simulink model "ASK_coerente"  (R2020a)
settings: Solver=VariableStepAuto  StartTime=0.0  StopTime=tsim  RelTol=1e-3
values from neighbouring files (symbols this model uses):
  Ac = 1    [init_vars.m]
  fc = 10e3    (= 10000)    [init_vars.m]
  fs = spb*rb    (= 100000)    [init_vars.m]
  ganho_int = rb    (= 1000)    [init_vars.m]
  lim = 0.5/2    (= 0.25)    [parte3ASK.m]    (also in parte3BPSK.m = 0; parte4.m = 0.5)
  rb = 1e3    (= 1000)    [init_vars.m]
  rng_seed = 5    [init_vars.m]
  spb = 100    [init_vars.m]
libraries: dspswit3 x2, commrandsrc3 x1, commchan3 x1, commfilt2 x1, dspsigops x1
settings Model: Creator=pedro  LastModifiedBy=pedro

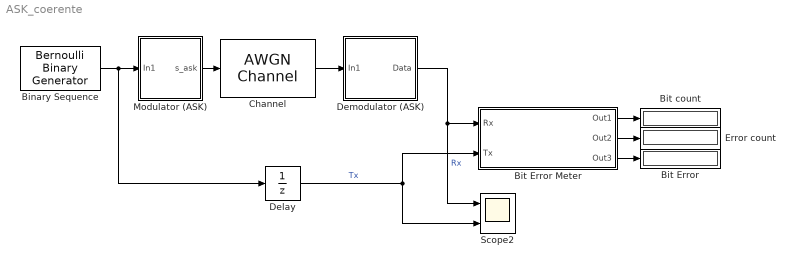
== system ASK_coerente ==
  Binary Sequence : commrandsrc3/Bernoulli Binary Generator  ProbabilityOfZero=0.5  SeedSource=Parameter  Seed=rng_seed  SampleTime=1/rb  SamplesPerFrame=1  OutputDataType=double  SimulateUsing=Interpreted execution
  Bit Error : Display
  Bit Error Meter : Subsystem
  Bit count : Display
  Channel : commchan3/AWGN Channel  InputProcessing=Columns as channels (frame based)  seed=rng_seed  noiseMode=Variance from mask  EbNodB=10  EsNodB=10  SNRdB=10  bitsPerSym=1  Ps=1  Tsym=1  variance=sigmaquadrado
  Delay : UnitDelay  SampleTime=1/rb  HasFrameUpgradeWarning=on
  Demodulator (ASK) : Subsystem
  Error count : Display
  Modulator (ASK) : Subsystem
  Scope2 : Scope  NumInputPorts=2
  wires:
  Binary Sequence/1 -> Delay/1, Modulator (ASK)/1(In1)
  Modulator (ASK)/1(s_ask) -> Channel/1
  Delay/1 -> Scope2/2, Bit Error Meter/2(Tx)  "Tx"
  Bit Error Meter/1(Out1) -> Bit count/1
  Bit Error Meter/2(Out2) -> Error count/1
  Bit Error Meter/3(Out3) -> Bit Error/1
  Demodulator (ASK)/1(Data) -> Bit Error Meter/1(Rx), Scope2/1  "Rx"
  Channel/1 -> Demodulator (ASK)/1(In1)

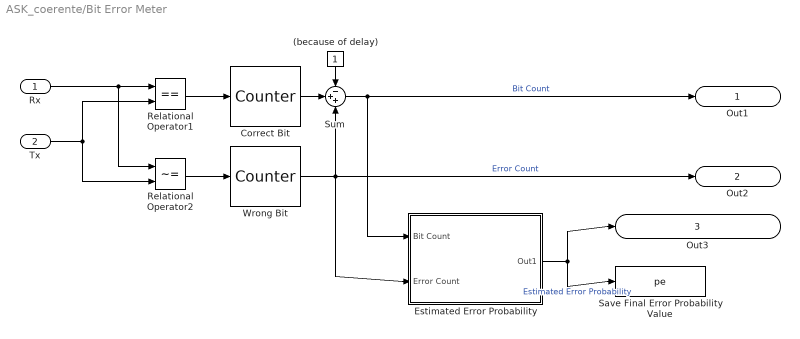
== system ASK_coerente/Bit Error Meter ==
  Rx : Inport
  Tx : Inport  Port=2
  (because of delay) : Constant
  Correct Bit : dspswit3/Counter  Direction=Up  CountEvent=Non-zero sample  CounterSize=32 bits  MaxCount=255  InitialCount=0  Output=Count  HitValue=32  ResetInput=off  SamplesPerFrame=1  Ts=1  CntDtype=uint32  HitDtype=Logical
  Estimated Error Probability : Subsystem
  Relational Operator1 : RelationalOperator  Operator===  OutDataTypeStr=boolean  RndMeth=Simplest
  Relational Operator2 : RelationalOperator  Operator=~=  OutDataTypeStr=boolean  RndMeth=Simplest
  Save Final Error Probability Value : ToWorkspace  VariableName=pe  SampleTime=-1
      settings: MaxDataPoints=1
  Sum : Sum  Inputs=-++
  Wrong Bit : dspswit3/Counter  Direction=Up  CountEvent=Non-zero sample  CounterSize=32 bits  MaxCount=255  InitialCount=0  Output=Count  HitValue=32  ResetInput=off  SamplesPerFrame=1  Ts=1  CntDtype=uint32  HitDtype=Logical
  Out1 : Outport
  Out2 : Outport  Port=2
  Out3 : Outport  Port=3
  wires:
  Relational Operator1/1 -> Correct Bit/1
  Correct Bit/1 -> Sum/2
  Rx/1 -> Relational Operator2/1, Relational Operator1/1
  Relational Operator2/1 -> Wrong Bit/1
  Sum/1 -> Estimated Error Probability/1(Bit Count), Out1/1  "Bit Count"
  Tx/1 -> Relational Operator2/2, Relational Operator1/2
  Wrong Bit/1 -> Estimated Error Probability/2(Error Count), Sum/3, Out2/1  "Error Count"
  (because of delay)/1 -> Sum/1
  Estimated Error Probability/1(Out1) -> Out3/1, Save Final Error Probability Value/1  "Estimated Error Probability"

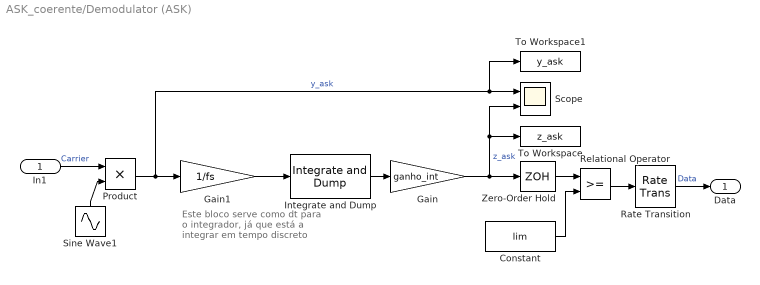
== system ASK_coerente/Demodulator (ASK) ==
  note: Este bloco serve como dt
      | para o integrador, já que está a integrar em tempo discreto
  In1 : Inport
  Constant : Constant  Value=lim
  Gain : Gain  Gain=ganho_int
  Gain1 : Gain  Gain=1/fs
  Integrate and Dump : commfilt2/Integrate and Dump  obssamples=spb  offsetsamples=1  nodump=on  roundingMode=Floor  overflowMode=off  outputDataTypeStr=Inherit: Same as accumulator  outputLastDataTypeStr=Inherit: Same as accumulator
  Product : Product
  Rate Transition : RateTransition  Integrity=off  OutPortSampleTime=1/rb
  Relational Operator : RelationalOperator  OutDataTypeStr=boolean  RndMeth=Simplest
  Scope : Scope  NumInputPorts=2
  Sine Wave1 : Sin  Amplitude=Ac  Frequency=2*pi*fc  SampleTime=1/fs
  To Workspace : ToWorkspace  VariableName=z_ask  SaveFormat=Timeseries  SampleTime=-1
  To Workspace1 : ToWorkspace  VariableName=y_ask  SaveFormat=Timeseries  SampleTime=-1
  Zero-Order Hold : ZeroOrderHold  SampleTime=1/rb
  Data : Outport
  wires:
  In1/1 -> Product/1  "Carrier"
  Product/1 -> To Workspace1/1, Scope/1, Gain1/1  "y_ask"
  Relational Operator/1 -> Rate Transition/1
  Sine Wave1/1 -> Product/2
  Integrate and Dump/1 -> Gain/1
  Constant/1 -> Relational Operator/2
  Zero-Order Hold/1 -> Relational Operator/1
  Gain/1 -> Scope/2, To Workspace/1, Zero-Order Hold/1  "z_ask"
  Rate Transition/1 -> Data/1  "Data"
  Gain1/1 -> Integrate and Dump/1

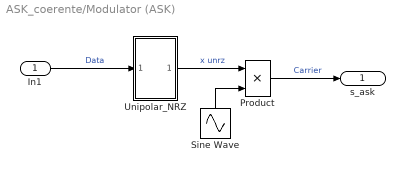
== system ASK_coerente/Modulator (ASK) ==
  In1 : Inport
  Product : Product
  Sine Wave : Sin  Amplitude=Ac  Frequency=2*pi*fc  SampleTime=1/fs
  Unipolar_NRZ : Subsystem  mask(unipolar_nrz){Rb=rb, Spb=spb}
      mask prompts: Rb "Binary Data Rate"; Spb "Samples per bit"
  s_ask : Outport
  wires:
  Sine Wave/1 -> Product/2
  Product/1 -> s_ask/1  "Carrier"
  Unipolar_NRZ/1(Out1) -> Product/1  "x unrz"
  In1/1 -> Unipolar_NRZ/1(In1)  "Data"

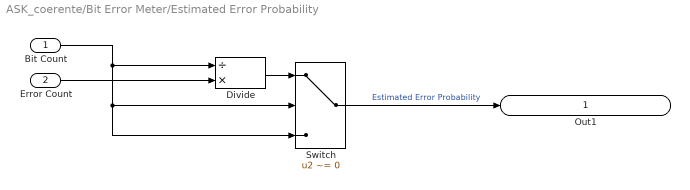
== system ASK_coerente/Bit Error Meter/Estimated Error Probability ==
  Bit Count : Inport
  Error Count : Inport  Port=2
  Divide : Product  Inputs=/*  OutDataTypeStr=double
  Switch : Switch  Criteria=u2 ~= 0
  Out1 : Outport
  wires:
  Bit Count/1 -> Divide/1, Switch/3, Switch/2
  Switch/1 -> Out1/1  "Estimated Error Probability"
  Divide/1 -> Switch/1
  Error Count/1 -> Divide/2

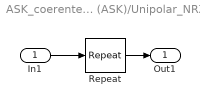
== system ASK_coerente/Modulator (ASK)/Unipolar_NRZ ==
  In1 : Inport
  Repeat : dspsigops/Repeat  N=Spb  InputProcessing=Columns as channels (frame based)  RateOptions=Allow multirate processing  ic=0  mode=Unused parameter value
  Out1 : Outport
  wires:
  In1/1 -> Repeat/1
  Repeat/1 -> Out1/1
